simulink model "velocity_subsystem_eso"  (R2019b)
settings: Solver=VariableStepAuto  StartTime=0.0  StopTime=100  RelTol=1e-3
values from neighbouring files (symbols this model uses):
  A = diag(ones(length(a)-2,1),1)    [eso_design.m]    (also in eso_design_angular_rate.m = [0 1 0; 0 0 1; 0 0 -500 ]; eso_design_velocity.m = diag(ones(size,1),1); tf2CCF.m; tf2ControlCanonical.m)
  B = zeros(length(a)-1,1)    [eso_design.m]    (also in eso_design_angular_rate.m = [0;B_CONTROL_SYS(end);-500*B_CONTROL_SYS(end)]; eso_design_velocity.m = zeros(size+1,1); tf2CCF.m = zeros(length(A),1))
  C = [1 0 0]    [eso_design_angular_rate.m]    (also in eso_design_velocity.m = zeros(1,size+1); tf2CCF.m = zeros(1,length(b)-1); tf2ControlCanonical.m = zeros(1,length(b)-1))
  G__V_N_PX4 = G__q2_PX4_CL*(4*Tmax/m)*(1/s)    [discrete_eso_design_velocity.m]    (also in eso_design.m; eso_design_velocity.m)
  L = acker(A',C',poles_eso)'    [eso_design.m]    (also in eso_design_angular_rate.m = [3*wd 3*wd^2 wd^3]'; eso_design_velocity.m = acker(A',C',eso_poles)')
undefined symbols (not defined in the file or in its folder): MPC_XY_VEL_D, MPC_XY_VEL_I, MPC_XY_VEL_P
libraries: simulink x1
settings Model: Creator=henry  LastModifiedBy=henry

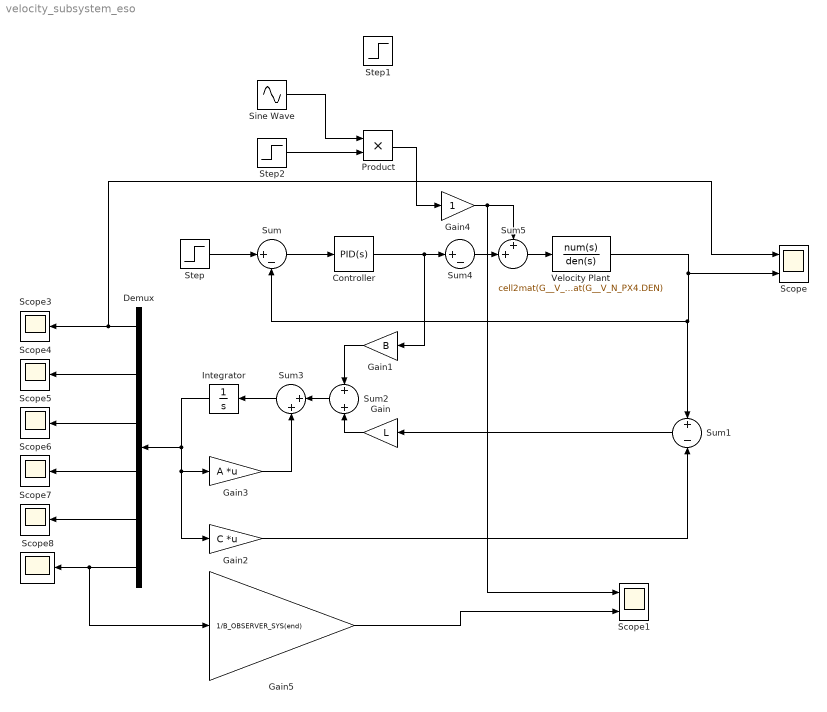
== system velocity_subsystem_eso ==
  Controller : simulink/Continuous/PID Controller  Controller=PID  Form=Ideal  TimeDomain=Continuous-time  SampleTime=-1  IntegratorMethod=Forward Euler  FilterMethod=Forward Euler  ControllerParametersSource=internal  P=MPC_XY_VEL_P  I=MPC_XY_VEL_I  D=MPC_XY_VEL_D  UseFilter=on  N=100  TunerSelectOption=Transfer Function Based (PID Tuner App)  InitialConditionSource=internal  InitialConditionForIntegrator=0  InitialConditionForFilter=0  DifferentiatorICPrevScaledInput=0  ExternalReset=none  TrackingMode=off  Kt=1  LimitOutput=off  UpperSaturationLimit=inf  LowerSaturationLimit=-inf  LinearizeAsGain=on  AntiWindupMode=none  Kb=1  POutMin=[]  POutMax=[]  IOutMin=[]  IOutMax=[]  DOutMin=[]  DOutMax=[]  NOutMin=[]  NOutMax=[]  SumOutMin=[]  SumOutMax=[]  SaturationOutMin=[]  SaturationOutMax=[]  PParamMin=[]  PParamMax=[]  IParamMin=[]  IParamMax=[]  DParamMin=[]  DParamMax=[]  NParamMin=[]  NParamMax=[]  KbParamMin=[]  KbParamMax=[]  KtParamMin=[]  KtParamMax=[]  KbOutMin=[]  KbOutMax=[]  KtOutMin=[]  KtOutMax=[]  IntegratorOutMin=[]  IntegratorOutMax=[]  FilterOutMin=[]  FilterOutMax=[]  SumI1OutMin=[]  SumI1OutMax=[]  SumI2OutMin=[]  SumI2OutMax=[]  SumI3OutMin=[]  SumI3OutMax=[]  SumI4OutMin=[]  SumI4OutMax=[]  SumDOutMin=[]  SumDOutMax=[]  DifferentiatorOutMin=[]  DifferentiatorOutMax=[]  FilterDiffOutCoefMin=[]  FilterDiffOutCoefMax=[]  ReciprocalOutMin=[]  ReciprocalOutMax=[]  SumDenOutMin=[]  SumDenOutMax=[]  SumNumOutMin=[]  SumNumOutMax=[]  DivideOutMin=[]  DivideOutMax=[]  IntegratorContinuousStateAttributes=''  IntegratorStateMustResolveToSignalObject=off  IntegratorRTWStateStorageClass=Auto  FilterContinuousStateAttributes=''  FilterStateMustResolveToSignalObject=off  FilterRTWStateStorageClass=Auto  ParallelPVariant=Passthrough  IdealPVariant=InternalParameters  IVariant=InternalParameters  DVariant=InternalParameters  IntegratorVariant=Continuous  SatVariant=Disabled  AWVariant=Passthrough  PCopyVariant=Disabled  TRVariant=Disabled  FdbkBlocksVariant=Forward  IdealPFdbkVariant=Disabled  SatFdbkVariant=Disabled  DerivativeFilterVariant=ContFilter  NVariant=InternalParameters  NCopyVariant=Disabled  FilterICVariant=InternalICsFilter  IntegratorICVariant=InternalICs  ExternalResetVariant=Disabled  TRSumVariant=Passthrough  SumFdbkVariant=Disabled  SumVariant=Sum_PID
  Demux : Demux  Outputs=6
  Gain : Gain  Gain=L
  Gain1 : Gain  Gain=B
  Gain2 : Gain  Gain=C  Multiplication=Matrix(K*u)
  Gain3 : Gain  Gain=A  Multiplication=Matrix(K*u)
  Gain4 : Gain
  Gain5 : Gain  Gain=1/B_OBSERVER_SYS(end)
  Integrator : Integrator
  Product : Product
  Scope : Scope  NumInputPorts=2
  Scope1 : Scope  NumInputPorts=2
  Scope{3..8} (6 alike) : Scope
  Sine Wave : Sin  Amplitude=0.01  SampleTime=0
  Step : Step  SampleTime=0
  Step1 : Step  Time=5  After=0.01  SampleTime=0
  Step2 : Step  Time=10  SampleTime=0
  Sum : Sum  Inputs=|+-
  Sum1 : Sum  Inputs=+|-
  Sum2 : Sum  Inputs=+|+
  Sum3 : Sum  Inputs=|++
  Sum4 : Sum  Inputs=|+-
  Sum5 : Sum  Inputs=++|
  Velocity Plant : TransferFcn  Numerator=cell2mat(G__V_N_PX4.NUM)  Denominator=cell2mat(G__V_N_PX4.DEN)
  wires:
  Controller/1 -> Gain1/1, Sum4/1
  Velocity Plant/1 -> Scope/2, Sum/2, Sum1/1
  Sum/1 -> Controller/1
  Step/1 -> Sum/1
  Sum1/1 -> Gain/1
  Gain1/1 -> Sum2/1
  Gain/1 -> Sum2/2
  Sum2/1 -> Sum3/1
  Sum3/1 -> Integrator/1
  Integrator/1 -> Gain2/1, Gain3/1, Demux/1
  Gain3/1 -> Sum3/2
  Demux/2 -> Scope4/1
  Demux/3 -> Scope5/1
  Demux/4 -> Scope6/1
  Demux/5 -> Scope7/1
  Demux/6 -> Gain5/1, Scope8/1
  Gain2/1 -> Sum1/2
  Sum4/1 -> Sum5/2
  Sum5/1 -> Velocity Plant/1
  Gain4/1 -> Scope1/1, Sum5/1
  Demux/1 -> Scope/1, Scope3/1
  Gain5/1 -> Scope1/2
  Product/1 -> Gain4/1
  Step2/1 -> Product/2
  Sine Wave/1 -> Product/1
